simulink model "P1_Week1_Deliverables"  (R2023b)
settings: Solver=ode1  StartTime=0.0  StopTime=25  FixedStep=0.1  RelTol=1e-3
values from neighbouring files (symbols this model uses):
  A = 1    [P1_Week1_Delieverables.m]
  b = 1    [P1_Week1_Delieverables.m]
  J = 1    [P1_Week1_Delieverables.m]
  w_0 = 1.0    (= 1)    [P1_Week1_Delieverables.m]
settings Model: Creator=dxego  LastModifiedBy=rafae

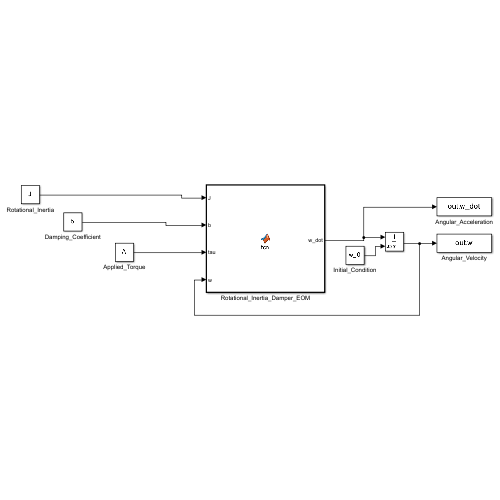
[thumbnail: Simulink's stored preview of the top-level diagram]
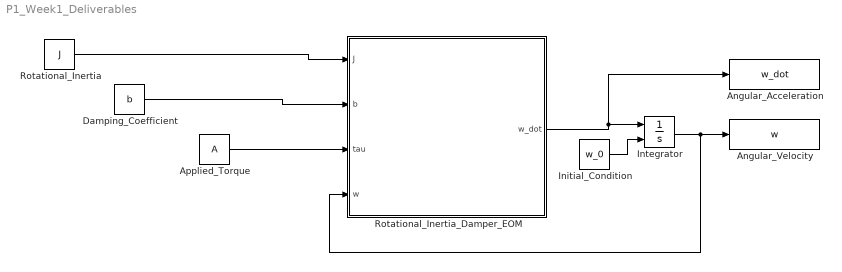
== system P1_Week1_Deliverables ==
  Angular_Acceleration : ToWorkspace  VariableName=w_dot  SaveFormat=Timeseries  SampleTime=-1
  Angular_Velocity : ToWorkspace  VariableName=w  SaveFormat=Timeseries  SampleTime=-1
  Applied_Torque : Constant  Value=A
  Damping_Coefficient : Constant  Value=b
  Initial_Condition : Constant  Value=w_0
  Integrator : Integrator  InitialConditionSource=external
  Rotational_Inertia : Constant  Value=J
  Rotational_Inertia_Damper_EOM : MATLAB Function  TreatAsAtomicUnit=on
  wires:
  Rotational_Inertia/1 -> Rotational_Inertia_Damper_EOM/1(J)
  Damping_Coefficient/1 -> Rotational_Inertia_Damper_EOM/2(b)
  Applied_Torque/1 -> Rotational_Inertia_Damper_EOM/3(tau)
  Rotational_Inertia_Damper_EOM/1(w_dot) -> Angular_Acceleration/1, Integrator/1
  Integrator/1 -> Rotational_Inertia_Damper_EOM/4(w), Angular_Velocity/1
  Initial_Condition/1 -> Integrator/2

== matlab function P1_Week1_Deliverables/Rotational_Inertia_Damper_EOM ==
  data: J input; w_dot output; b input; tau input; w input
function w_dot = fcn(J, b, tau, w)
% Recall EOM: J*w_dot = tau_applied - tau_damped
tau_damped = b*w;
w_dot = (1/J)*(tau - tau_damped);
end
